simulink model "cruise_control"  (R2018a)
settings: Solver=VariableStepAuto  StartTime=0.0  StopTime=120  RelTol=1e-3
values from neighbouring files (symbols this model uses):
  b = 3.5077E-6    (= 3.5077e-06)    [DC_motor_position.m]    (also in DC_motor_speed_para.m = 0.1; cruise_control_para.m = 50)
  ki = 40    [cruise_control_para.m]
  kp = 800    [cruise_control_para.m]
  m = 1000    [cruise_control_para.m]
  r = 500    [cruise_control_para.m]
settings Model: Creator=Infi  LastModifiedBy=Infi

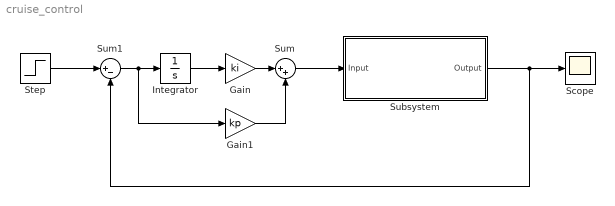
== system cruise_control ==
  Gain : Gain  Gain=ki
  Gain1 : Gain  Gain=kp
  Integrator : Integrator
  Scope : Scope
  Step : Step  After=r  SampleTime=0
  Subsystem : Subsystem
  Sum : Sum  Inputs=|++
  Sum1 : Sum  Inputs=|+-
  wires:
  Sum/1 -> Subsystem/1(Input)
  Subsystem/1(Output) -> Sum1/2, Scope/1
  Step/1 -> Sum1/1
  Sum1/1 -> Gain1/1, Integrator/1
  Integrator/1 -> Gain/1
  Gain/1 -> Sum/1
  Gain1/1 -> Sum/2

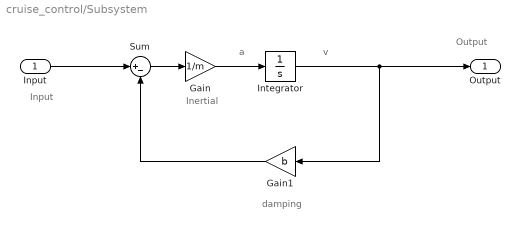
== system cruise_control/Subsystem ==
  note: Output
  note: Input
  note: v
  note: a
  note: damping
  note: Inertial
  Input : Inport
  Gain : Gain  Gain=1/m
  Gain1 : Gain  Gain=b
  Integrator : Integrator
  Sum : Sum  Inputs=|+-
  Output : Outport
  wires:
  Sum/1 -> Gain/1
  Input/1 -> Sum/1
  Gain/1 -> Integrator/1
  Integrator/1 -> Output/1, Gain1/1
  Gain1/1 -> Sum/2
